simulink model "fw_att_control"  (R2021a)
settings: Solver=FixedStepAuto  StartTime=0.0  StopTime=10.0  RelTol=1e-3
undefined symbols (not defined in the file): DiscIntNeverNeededParam, FW_ACRO_X_MAX, FW_ACRO_Y_MAX, FW_ACRO_Z_MAX, FW_AIRSPD_MAX, FW_AIRSPD_STALL, FW_AIRSPD_TRIM, FW_BAT_SCALE_EN, FW_DTRIM_P_FLPS, FW_DTRIM_P_VMAX, FW_DTRIM_P_VMIN, FW_DTRIM_R_FLPS, FW_DTRIM_R_VMAX, FW_DTRIM_R_VMIN, FW_DTRIM_Y_VMAX, FW_DTRIM_Y_VMIN, FW_FLAPERON_SCL, FW_FLAPS_LND_SCL, FW_FLAPS_SCL, FW_FLAPS_TO_SCL, FW_MAN_P_MAX, FW_MAN_P_SC, FW_MAN_R_MAX, FW_MAN_R_SC, FW_MAN_Y_SC, FW_P_TC, FW_PR_IMAX, FW_PR_P, FW_PSP_OFF, FW_R_TC, FW_RLL_TO_YAW_FF, FW_RR_FF, FW_W_EN, FW_W_RMAX, FW_WR_FF, FW_WR_P, FW_Y_TC, FW_YR_FF, FW_YR_P, magnitude, PX4_VEHICLE_ATTITUDE_SETPOINT, PX4_VEHICLE_STATUS, TRIM_PITCH, TRIM_ROLL, TRIM_YAW
libraries: simulink x10, aerolibconvert2 x5, sharedtransform x2
(part 1 of 2)
settings Model: DataDictionary=px4_dict.sldd  Creator=DELL  LastModifiedBy=DELL
settings OptimizationCC: DefaultUnderspecifiedDataType=single

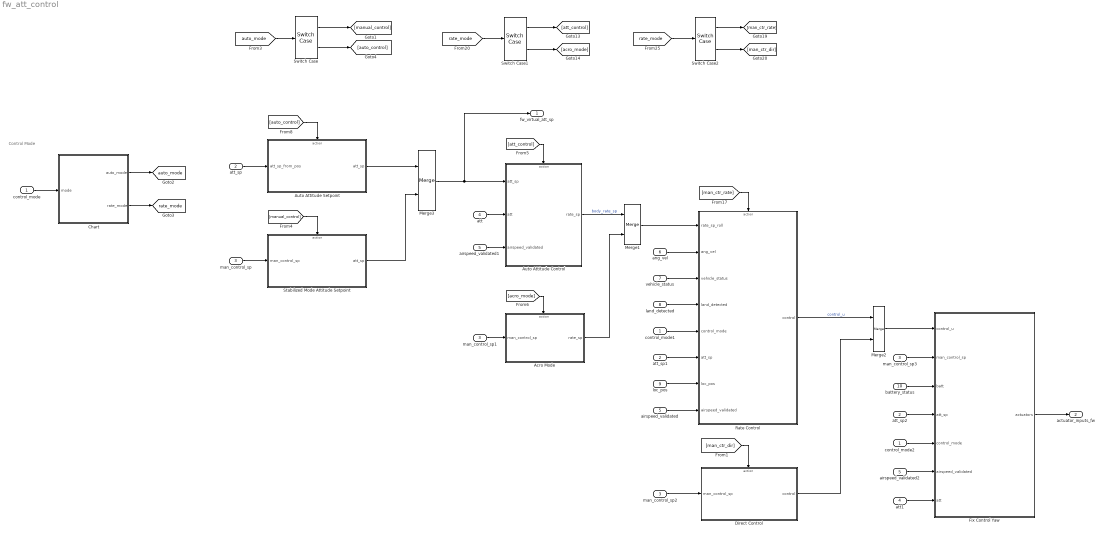
== system fw_att_control ==
  note: Control Mode
  control_mode : Inport  OutDataTypeStr=Bus: px4_vehicle_control_mode  BusOutputAsStruct=on
  att_sp : Inport  Port=2  OutDataTypeStr=Bus: px4_vehicle_attitude_setpoint  BusOutputAsStruct=on
  man_control_sp2 : Inport  Port=3  OutDataTypeStr=Bus: px4_manual_control_setpoint  BusOutputAsStruct=on
  att : Inport  Port=4  OutDataTypeStr=Bus: px4_vehicle_attitude  BusOutputAsStruct=on
  airspeed_validated1 : Inport  Port=5  OutDataTypeStr=Bus: px4_airspeed_validated  BusOutputAsStruct=on
  ang_vel : Inport  Port=6  OutDataTypeStr=Bus: px4_vehicle_angular_velocity  BusOutputAsStruct=on
  vehicle_status : Inport  Port=7  OutDataTypeStr=Bus: px4_vehicle_status  BusOutputAsStruct=on
  land_detected : Inport  Port=8  OutDataTypeStr=Bus: px4_vehicle_land_detected  BusOutputAsStruct=on
  loc_pos : Inport  Port=9  OutDataTypeStr=Bus: px4_vehicle_local_position
  battery_status : Inport  Port=10  OutDataTypeStr=Bus: px4_battery_status  BusOutputAsStruct=on
  Acro Mode : Subsystem  TreatAsAtomicUnit=on
  Auto Attitude Control : Subsystem
  Auto Attitude Setpoint : Subsystem
  Chart : Stateflow chart  TreatAsAtomicUnit=on
  "Direct Control " : Subsystem  TreatAsAtomicUnit=on
  Fix Control Yaw : Subsystem
  Merge1 : Merge
  Merge2 : Merge
  Merge3 : Merge
  Rate Control : Subsystem
  Stabilized Mode Attitude Setpoint : Subsystem  TreatAsAtomicUnit=on
  Switch Case : SwitchCase  CaseConditions={1,2 }  ShowDefaultCase=off
  Switch Case1 : SwitchCase  CaseConditions={1,2}  ShowDefaultCase=off
  Switch Case2 : SwitchCase  CaseConditions={2}
  airspeed_validated : InportShadow  Port=5  OutDataTypeStr=Bus: px4_airspeed_validated  BusOutputAsStruct=on
  airspeed_validated2 : InportShadow  Port=5  OutDataTypeStr=Bus: px4_airspeed_validated  BusOutputAsStruct=on
  att1 : InportShadow  Port=4  OutDataTypeStr=Bus: px4_vehicle_attitude  BusOutputAsStruct=on
  att_sp1 : InportShadow  Port=2  OutDataTypeStr=Bus: px4_vehicle_attitude_setpoint  BusOutputAsStruct=on
  att_sp2 : InportShadow  Port=2  OutDataTypeStr=Bus: px4_vehicle_attitude_setpoint  BusOutputAsStruct=on
  control_mode1 : InportShadow  OutDataTypeStr=Bus: px4_vehicle_control_mode  BusOutputAsStruct=on
  control_mode2 : InportShadow  OutDataTypeStr=Bus: px4_vehicle_control_mode  BusOutputAsStruct=on
  man_control_sp : InportShadow  Port=3  OutDataTypeStr=Bus: px4_manual_control_setpoint  BusOutputAsStruct=on
  man_control_sp1 : InportShadow  Port=3  OutDataTypeStr=Bus: px4_manual_control_setpoint  BusOutputAsStruct=on
  man_control_sp3 : InportShadow  Port=3  OutDataTypeStr=Bus: px4_manual_control_setpoint  BusOutputAsStruct=on
  fw_virtual_att_sp : Outport  OutDataTypeStr=Bus: px4_vehicle_attitude_setpoint  BusOutputAsStruct=on
  actuator_inputs_fw : Outport  Port=2  OutDataTypeStr=Bus: px4_actuator_controls_0  BusOutputAsStruct=on
  tag scope: auto_mode=global, rate_mode=global
  wires:
  Chart/1(auto_mode) -> [auto_mode]
  Chart/2(rate_mode) -> [rate_mode]
  control_mode/1 -> Chart/1(mode)
  att_sp2/1 -> Fix Control Yaw/4(att_sp)
  Auto Attitude Control/1(rate_sp) -> Merge1/1  "body_rate_sp"
  Acro Mode/1(rate_sp) -> Merge1/2
  [att_control] -> Auto Attitude Control/Action
  Switch Case1/2 -> [acro_mode]
  att/1 -> Auto Attitude Control/2(att)
  [rate_mode] -> Switch Case1/1
  Switch Case1/1 -> [att_control]
  man_control_sp1/1 -> Acro Mode/1(man_control_sp)
  Merge2/1 -> Fix Control Yaw/1(control_u)
  Rate Control/1(control) -> Merge2/1  "control_u"
  ang_vel/1 -> Rate Control/2(ang_vel)
  "Direct Control "/1(control) -> Merge2/2
  Switch Case2/2 -> [man_ctr_dir]
  [man_ctr_dir] -> "Direct Control "/Action
  [man_ctr_rate] -> Rate Control/Action
  Switch Case2/1 -> [man_ctr_rate]
  [rate_mode] -> Switch Case2/1
  man_control_sp2/1 -> "Direct Control "/1(man_control_sp)
  man_control_sp3/1 -> Fix Control Yaw/2(man_control_sp)
  control_mode2/1 -> Fix Control Yaw/5(control_mode)
  vehicle_status/1 -> Rate Control/3(vehicle_status)
  land_detected/1 -> Rate Control/4(land_detected)
  control_mode1/1 -> Rate Control/5(control_mode)
  att_sp1/1 -> Rate Control/6(att_sp)
  battery_status/1 -> Fix Control Yaw/3(batt)
  Merge1/1 -> Rate Control/1(rate_sp_roll)
  airspeed_validated2/1 -> Fix Control Yaw/6(airspeed_validated)
  airspeed_validated1/1 -> Auto Attitude Control/3(airspeed_validated)
  airspeed_validated/1 -> Rate Control/8(airspeed_validated)
  loc_pos/1 -> Rate Control/7(loc_pos)
  [auto_mode] -> Switch Case/1
  [acro_mode] -> Acro Mode/Action
  Switch Case/1 -> [manual_control]
  Switch Case/2 -> [auto_control]
  man_control_sp/1 -> Stabilized Mode Attitude Setpoint/1(man_control_sp)
  Merge3/1 -> fw_virtual_att_sp/1, Auto Attitude Control/1(att_sp)
  [manual_control] -> Stabilized Mode Attitude Setpoint/Action
  [auto_control] -> Auto Attitude Setpoint/Action
  att1/1 -> Fix Control Yaw/7(att)
  Fix Control Yaw/1(actuators) -> actuator_inputs_fw/1
  Stabilized Mode Attitude Setpoint/1(att_sp) -> Merge3/2
  Auto Attitude Setpoint/1(att_sp) -> Merge3/1
  att_sp/1 -> Auto Attitude Setpoint/1(att_sp_from_pos)

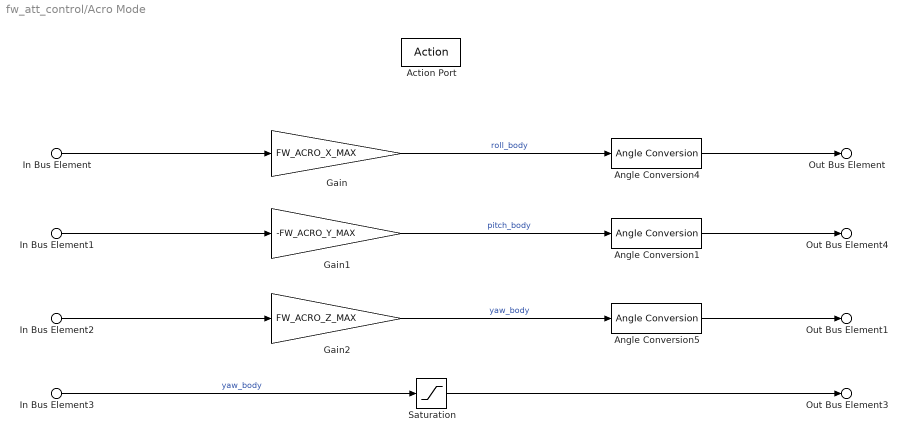
== system fw_att_control/Acro Mode ==
  In Bus Element : Inport  PortName=man_control_sp  Element=y
  In Bus Element1 : Inport  PortName=man_control_sp  Element=x
  In Bus Element2 : Inport  PortName=man_control_sp  Element=r
  In Bus Element3 : Inport  PortName=man_control_sp  Element=z
  Action Port : ActionPort  ActionPortLabel=case [ 2 ]:
  Angle Conversion1 : aerolibconvert2/Angle Conversion  IU=deg  OU=rad
  Angle Conversion4 : aerolibconvert2/Angle Conversion  IU=deg  OU=rad
  Angle Conversion5 : aerolibconvert2/Angle Conversion  IU=deg  OU=rad
  Gain : Gain  Gain=FW_ACRO_X_MAX
  Gain1 : Gain  Gain=-FW_ACRO_Y_MAX
  Gain2 : Gain  Gain=FW_ACRO_Z_MAX
  Saturation : Saturate  UpperLimit=1  LowerLimit=0
      settings: AttributesFormatString=[%<LowerLimit>,%<UpperLimit>]
  Out Bus Element : Outport  PortName=rate_sp  Element=roll
  Out Bus Element4 : Outport  PortName=rate_sp  Element=pitch
  Out Bus Element1 : Outport  PortName=rate_sp  Element=yaw
  Out Bus Element3 : Outport  PortName=rate_sp  Element=thrust
  wires:
  Gain1/1 -> Angle Conversion1/1  "pitch_body"
  In Bus Element3/1 -> Saturation/1  "yaw_body"
  Gain/1 -> Angle Conversion4/1  "roll_body"
  In Bus Element/1 -> Gain/1
  In Bus Element1/1 -> Gain1/1
  In Bus Element2/1 -> Gain2/1
  Gain2/1 -> Angle Conversion5/1  "yaw_body"
  Saturation/1 -> Out Bus Element3/1
  Angle Conversion4/1 -> Out Bus Element/1
  Angle Conversion1/1 -> Out Bus Element4/1
  Angle Conversion5/1 -> Out Bus Element1/1

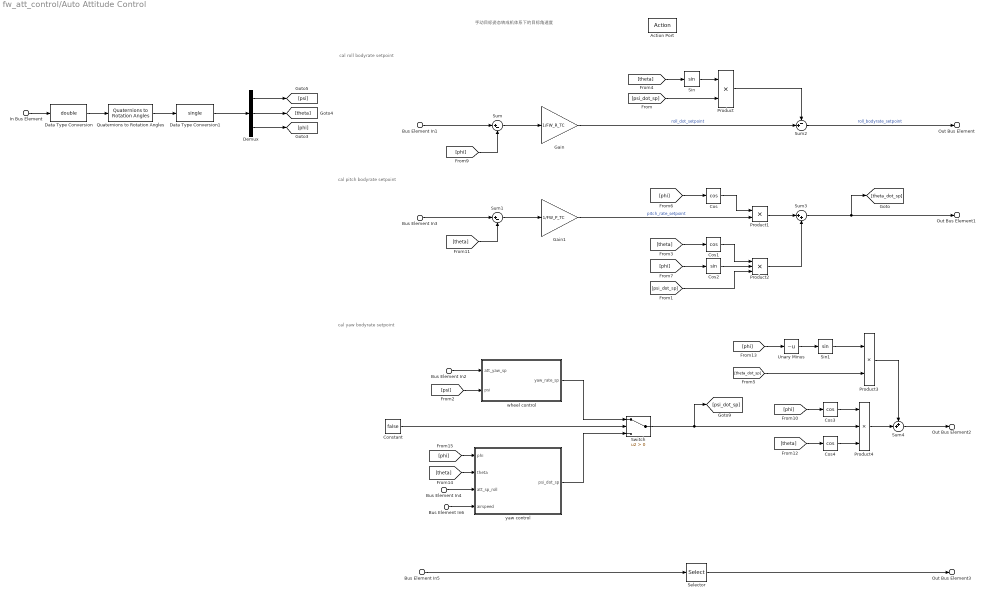
== system fw_att_control/Auto Attitude Control ==
  note: cal yaw bodyrate setpoint
  note: cal pitch bodyrate setpoint
  note: cal roll bodyrate setpoint
  note: 手动目标姿态转成机体系下的目标角速度
  Bus Element In3 : Inport  PortName=att_sp  Element=pitch_body
  Bus Element In5 : Inport  PortName=att_sp  Element=thrust_body
  Bus Element In2 : Inport  PortName=att_sp  Element=yaw_body
  Bus Element In1 : Inport  PortName=att_sp  Element=roll_body
  Bus Element In4 : Inport  PortName=att_sp  Element=roll_body
  In Bus Element : Inport  Port=2  PortName=att  Element=q
  Bus Element In6 : Inport  Port=3  PortName=airspeed_validated  Element=calibrated_airspeed_m_s
  Action Port : ActionPort  ActionPortLabel=case [ 1 ]:
  Constant : Constant  Value=false  OutDataTypeStr=boolean
  Cos{,1,3..4} (4 alike) : Trigonometry  Operator=cos
  Cos2 : Trigonometry
  Data Type Conversion : DataTypeConversion  OutDataTypeStr=double
  Data Type Conversion1 : DataTypeConversion  OutDataTypeStr=single
  Demux : Demux  Outputs=3
  Gain : Gain  Gain=1/FW_R_TC
  Gain1 : Gain  Gain=1/FW_P_TC
  Product : Product
  Product1 : Product
  Product2 : Product  Inputs=3
  Product3 : Product
  Product4 : Product  Inputs=3
  Quaternions to Rotation Angles : sharedtransform/Quaternions to Rotation Angles  rotationOrder=ZYX  aMode=aMode
      settings: SourceProductBaseCode=AE,PW,DR,MT,UV,VE
  Selector : Selector  InputPortWidth=3  IndexOptions=Index vector (dialog)  Indices=[1]  OutputSizes=1
  Sin : Trigonometry
  Sin1 : Trigonometry
  Sum : Sum  Inputs=|+-
  Sum1 : Sum  Inputs=|+-
  Sum2 : Sum  Inputs=-+|
  Sum3 : Sum  Inputs=|++
  Sum4 : Sum  Inputs=++|
  Switch : Switch  Criteria=u2 > Threshold
  Unary Minus : UnaryMinus
  wheel control : Subsystem  TreatAsAtomicUnit=on
  yaw control : Subsystem  TreatAsAtomicUnit=on
  Out Bus Element : Outport  PortName=rate_sp  Element=roll
  Out Bus Element1 : Outport  PortName=rate_sp  Element=pitch
  Out Bus Element2 : Outport  PortName=rate_sp  Element=yaw
  Out Bus Element3 : Outport  PortName=rate_sp  Element=thrust
  wires:
  Quaternions to Rotation Angles/1 -> Data Type Conversion1/1
  In Bus Element/1 -> Data Type Conversion/1
  Data Type Conversion/1 -> Quaternions to Rotation Angles/1
  Data Type Conversion1/1 -> Demux/1
  Demux/1 -> [psi]
  Demux/2 -> [theta]
  Demux/3 -> [phi]
  Sum3/1 -> Out Bus Element1/1, [theta_dot_sp]
  Sum2/1 -> Out Bus Element/1  "roll_bodyrate_setpoint"
  [theta] -> Sin/1
  Sin/1 -> Product/1
  Sum/1 -> Gain/1
  [phi] -> Sum/2
  [psi_dot_sp] -> Product/2
  Gain/1 -> Sum2/2  "roll_dot_setpoint"
  Bus Element In1/1 -> Sum/1
  Product/1 -> Sum2/1
  Bus Element In3/1 -> Sum1/1
  Cos1/1 -> Product2/1
  Cos/1 -> Product1/1
  Cos2/1 -> Product2/2
  Product2/1 -> Sum3/2
  Sum1/1 -> Gain1/1
  Product1/1 -> Sum3/1
  [theta] -> Cos1/1
  [psi_dot_sp] -> Product2/3
  [theta] -> Sum1/2
  [phi] -> Cos/1
  Gain1/1 -> Product1/2  "pitch_rate_setpoint"
  [phi] -> Cos2/1
  Bus Element In5/1 -> Selector/1
  [phi] -> Cos3/1
  [phi] -> Unary Minus/1
  Switch/1 -> Product4/2, [psi_dot_sp]
  Unary Minus/1 -> Sin1/1
  [theta_dot_sp] -> Product3/2
  Bus Element In4/1 -> yaw control/3(att_sp_roll)
  Bus Element In6/1 -> yaw control/4(airspeed)
  [psi] -> wheel control/2(psi)
  Bus Element In2/1 -> wheel control/1(att_yaw_sp)
  Sum4/1 -> Out Bus Element2/1
  Cos3/1 -> Product4/1
  Product3/1 -> Sum4/1
  Product4/1 -> Sum4/2
  Sin1/1 -> Product3/1
  [theta] -> Cos4/1
  Cos4/1 -> Product4/3
  [phi] -> yaw control/1(phi)
  [theta] -> yaw control/2(theta)
  wheel control/1(yaw_rate_sp) -> Switch/1
  yaw control/1(psi_dot_sp) -> Switch/3
  Constant/1 -> Switch/2
  Selector/1 -> Out Bus Element3/1

== system fw_att_control/Auto Attitude Setpoint ==
  att_sp_from_pos : Inport
  Action Port : ActionPort  ActionPortLabel=case [ 2 ]:
  Signal Conversion : SignalConversion  ConversionOutput=Virtual bus  OverrideOpt=off
  att_sp : Outport
  wires:
  att_sp_from_pos/1 -> Signal Conversion/1
  Signal Conversion/1 -> att_sp/1

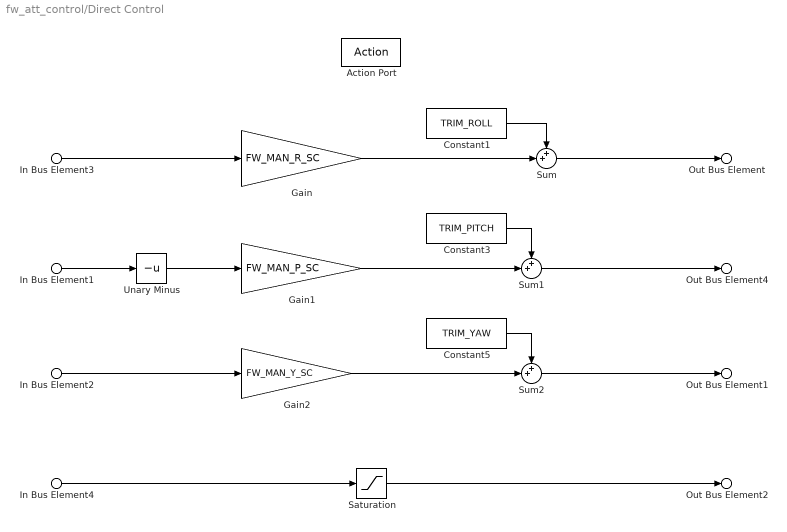
== system fw_att_control/Direct Control  ==
  In Bus Element3 : Inport  PortName=man_control_sp  Element=y
  In Bus Element1 : Inport  PortName=man_control_sp  Element=x
  In Bus Element2 : Inport  PortName=man_control_sp  Element=r
  In Bus Element4 : Inport  PortName=man_control_sp  Element=z
  Action Port : ActionPort  ActionPortLabel=default:
  Constant1 : Constant  Value=TRIM_ROLL
  Constant3 : Constant  Value=TRIM_PITCH
  Constant5 : Constant  Value=TRIM_YAW
  Gain : Gain  Gain=FW_MAN_R_SC
  Gain1 : Gain  Gain=FW_MAN_P_SC
  Gain2 : Gain  Gain=FW_MAN_Y_SC
  Saturation : Saturate  UpperLimit=1  LowerLimit=0
      settings: AttributesFormatString=[%<LowerLimit>,%<UpperLimit>]
  Sum : Sum  Inputs=++|
  Sum1 : Sum  Inputs=++|
  Sum2 : Sum  Inputs=++|
  Unary Minus : UnaryMinus
  Out Bus Element : Outport  PortName=control  Element=index_roll
  Out Bus Element4 : Outport  PortName=control  Element=index_pitch
  Out Bus Element1 : Outport  PortName=control  Element=index_yaw
  Out Bus Element2 : Outport  PortName=control  Element=index_throttle
  wires:
  In Bus Element3/1 -> Gain/1
  Sum/1 -> Out Bus Element/1
  Sum1/1 -> Out Bus Element4/1
  In Bus Element1/1 -> Unary Minus/1
  Unary Minus/1 -> Gain1/1
  In Bus Element2/1 -> Gain2/1
  Sum2/1 -> Out Bus Element1/1
  In Bus Element4/1 -> Saturation/1
  Saturation/1 -> Out Bus Element2/1
  Constant1/1 -> Sum/1
  Gain/1 -> Sum/2
  Constant3/1 -> Sum1/1
  Gain1/1 -> Sum1/2
  Constant5/1 -> Sum2/1
  Gain2/1 -> Sum2/2

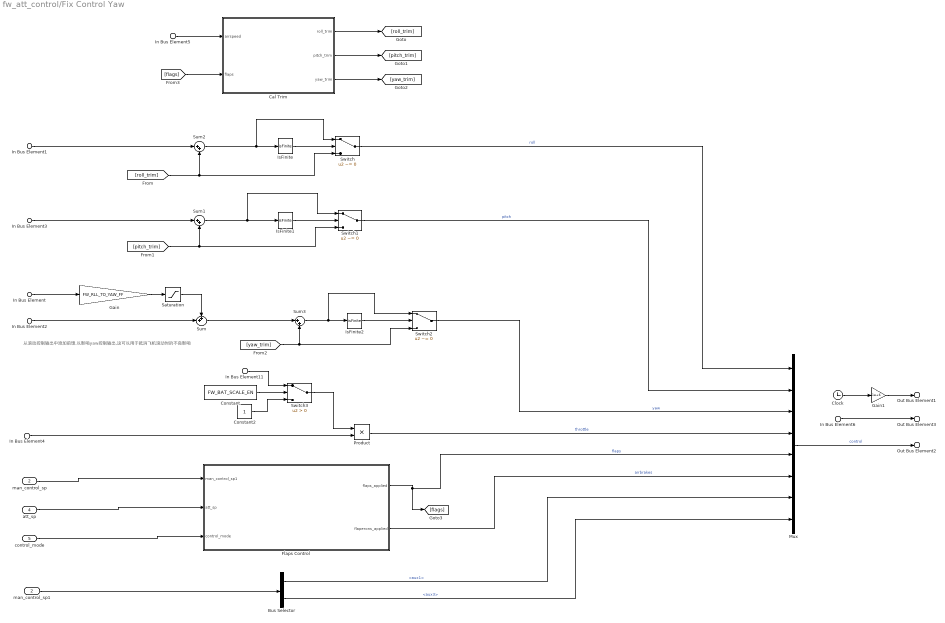
== system fw_att_control/Fix Control Yaw ==
  note: 从滚动控制输出中添加前馈,以影响yaw控制输出,这可以用于抵消飞机滚动时的不良影响
  In Bus Element1 : Inport  PortName=control_u  Element=index_roll
  In Bus Element : Inport  PortName=control_u  Element=index_roll
  In Bus Element3 : Inport  PortName=control_u  Element=index_pitch
  In Bus Element2 : Inport  PortName=control_u  Element=index_yaw
  In Bus Element4 : Inport  PortName=control_u  Element=index_throttle
  man_control_sp : Inport  Port=2
  In Bus Element11 : Inport  Port=3  PortName=batt  Element=scale
  att_sp : Inport  Port=4
  control_mode : Inport  Port=5
  In Bus Element5 : Inport  Port=6  PortName=airspeed_validated  Element=calibrated_airspeed_m_s
  In Bus Element6 : Inport  Port=7  PortName=att  Element=timestamp
  Bus Selector : BusSelector  OutputSignals=aux1,aux3
  Cal Trim : Subsystem
  Clock : Clock
  Constant : Constant  Value=FW_BAT_SCALE_EN  OutDataTypeStr=boolean
  Constant2 : Constant  OutDataTypeStr=single
  Flaps Control : Subsystem
  Gain : Gain  Gain=FW_RLL_TO_YAW_FF
  Gain1 : Gain  Gain=1e+6  OutDataTypeStr=uint64
      settings: AttributesFormatString=%<Gain>
  IsFinite : RelationalOperator  Operator=isFinite  OutDataTypeStr=boolean  RndMeth=Simplest
  IsFinite1 : RelationalOperator  Operator=isFinite  OutDataTypeStr=boolean  RndMeth=Simplest
  IsFinite2 : RelationalOperator  Operator=isFinite  OutDataTypeStr=boolean  RndMeth=Simplest
  Mux : Mux  Inputs=8
  Product : Product
  Saturation : Saturate  UpperLimit=1  LowerLimit=-1
      settings: AttributesFormatString=[%<LowerLimit>,%<UpperLimit>]
  Sum : Sum  Inputs=++|
  Sum1 : Sum  Inputs=|++
  Sum2 : Sum  Inputs=|++
  Sum3 : Sum  Inputs=|++
  Switch : Switch  Criteria=u2 ~= 0
  Switch1 : Switch  Criteria=u2 ~= 0
  Switch2 : Switch  Criteria=u2 ~= 0
  Switch3 : Switch  Criteria=u2 > Threshold
  man_control_sp1 : InportShadow  Port=2
  Out Bus Element1 : Outport  PortName=actuators  Element=timestamp
  Out Bus Element3 : Outport  PortName=actuators  Element=timestamp_sample
  Out Bus Element2 : Outport  PortName=actuators  Element=control
  wires:
  In Bus Element/1 -> Gain/1
  Saturation/1 -> Sum/1
  In Bus Element2/1 -> Sum/2
  Product/1 -> Mux/4  "throttle"
  control_mode/1 -> Flaps Control/3(control_mode)
  att_sp/1 -> Flaps Control/2(att_sp)
  Bus Selector/1 -> Mux/7  "<aux1>"
  Bus Selector/2 -> Mux/8  "<aux3>"
  Flaps Control/2(flaperons_applied) -> Mux/6  "airbrakes"
  man_control_sp/1 -> Flaps Control/1(man_control_sp1)
  Flaps Control/1(flaps_applied) -> Mux/5, [flags]  "flaps"
  man_control_sp1/1 -> Bus Selector/1
  In Bus Element4/1 -> Product/2
  In Bus Element1/1 -> Sum2/1
  Sum2/1 -> Switch/1, IsFinite/1
  IsFinite/1 -> Switch/2
  Switch/1 -> Mux/1  "roll"
  Switch1/1 -> Mux/2  "pitch"
  IsFinite1/1 -> Switch1/2
  IsFinite2/1 -> Switch2/2
  Switch2/1 -> Mux/3  "yaw"
  Sum/1 -> Sum3/1
  In Bus Element11/1 -> Switch3/1
  Constant/1 -> Switch3/2
  Switch3/1 -> Product/1
  Constant2/1 -> Switch3/3
  Sum1/1 -> Switch1/1, IsFinite1/1
  Sum3/1 -> Switch2/1, IsFinite2/1
  Cal Trim/1(roll_trim) -> [roll_trim]
  In Bus Element3/1 -> Sum1/1
  Cal Trim/2(pitch_trim) -> [pitch_trim]
  Cal Trim/3(yaw_trim) -> [yaw_trim]
  [pitch_trim] -> Switch1/3, Sum1/2
  [roll_trim] -> Sum2/2, Switch/3
  [yaw_trim] -> Sum3/2, Switch2/3
  [flags] -> Cal Trim/2(flaps)
  In Bus Element5/1 -> Cal Trim/1(airspeed)
  Gain/1 -> Saturation/1
  Clock/1 -> Gain1/1
  Gain1/1 -> Out Bus Element1/1
  Mux/1 -> Out Bus Element2/1  "control"
  In Bus Element6/1 -> Out Bus Element3/1

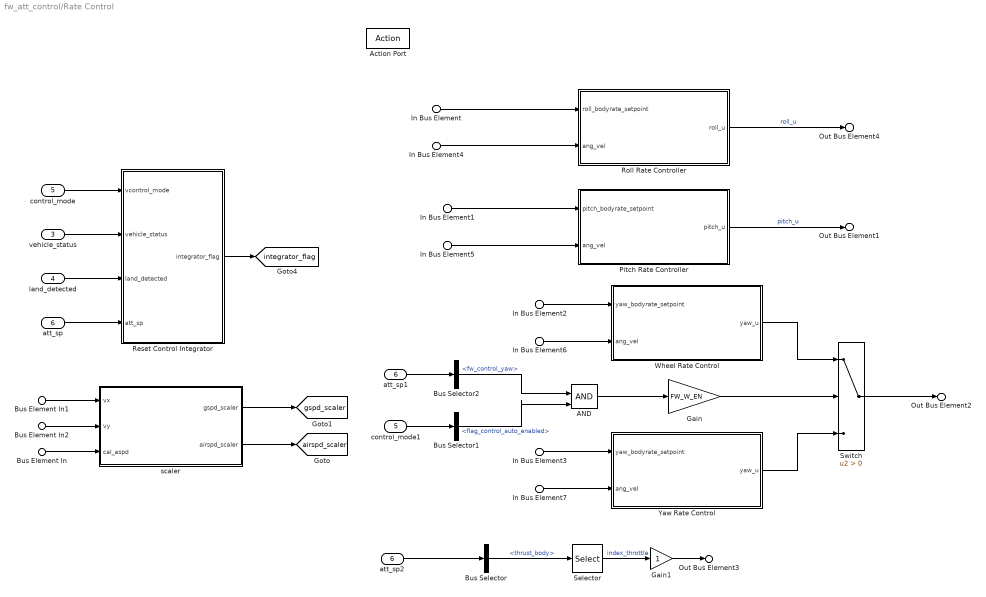
== system fw_att_control/Rate Control ==
  In Bus Element : Inport  PortName=rate_sp_roll  Element=roll
  In Bus Element1 : Inport  PortName=rate_sp_roll  Element=pitch
  In Bus Element2 : Inport  PortName=rate_sp_roll  Element=yaw
  In Bus Element3 : Inport  PortName=rate_sp_roll  Element=yaw
  In Bus Element{4..7} (4 alike) : Inport  Port=2  PortName=ang_vel  Element=xyz
  vehicle_status : Inport  Port=3  OutDataTypeStr=Bus: px4_vehicle_status
  land_detected : Inport  Port=4  OutDataTypeStr=Bus: px4_vehicle_land_detected
  control_mode : Inport  Port=5  OutDataTypeStr=Bus: px4_vehicle_control_mode
  att_sp : Inport  Port=6
  Bus Element In1 : Inport  Port=7  PortName=loc_pos  Element=vx
  Bus Element In2 : Inport  Port=7  PortName=loc_pos  Element=vy
  Bus Element In : Inport  Port=8  PortName=airspeed_validated  Element=calibrated_airspeed_m_s
  Action Port : ActionPort  ActionPortLabel=case [ 2 ]:
  AND : Logic  IconShape=distinctive  AllPortsSameDT=off  OutDataTypeStr=boolean
  Bus Selector : BusSelector  OutputSignals=thrust_body
  Bus Selector1 : BusSelector  OutputSignals=flag_control_auto_enabled
  Bus Selector2 : BusSelector  OutputSignals=fw_control_yaw
  Gain : Gain  Gain=FW_W_EN
  Gain1 : Gain
  Pitch Rate Controller : Subsystem
  Reset Control Integrator : Subsystem
  Roll Rate Controller : Subsystem
  Selector : Selector  InputPortWidth=3  IndexOptions=Index vector (dialog)  Indices=[1]  OutputSizes=1
  Switch : Switch  Criteria=u2 > Threshold
  Wheel Rate Control : Subsystem
  Yaw Rate Control : Subsystem
  att_sp1 : InportShadow  Port=6
  att_sp2 : InportShadow  Port=6
  control_mode1 : InportShadow  Port=5  OutDataTypeStr=Bus: px4_vehicle_control_mode
  scaler : Subsystem
  Out Bus Element4 : Outport  PortName=control  Element=index_roll
  Out Bus Element1 : Outport  PortName=control  Element=index_pitch
  Out Bus Element2 : Outport  PortName=control  Element=index_yaw
  Out Bus Element3 : Outport  PortName=control  Element=index_throttle
  tag scope: airspd_scaler=global, gspd_scaler=global, integrator_flag=global
  wires:
  In Bus Element/1 -> Roll Rate Controller/1(roll_bodyrate_setpoint)
  In Bus Element1/1 -> Pitch Rate Controller/1(pitch_bodyrate_setpoint)
  In Bus Element5/1 -> Pitch Rate Controller/2(ang_vel)
  Selector/1 -> Gain1/1  "index_throttle"
  vehicle_status/1 -> Reset Control Integrator/2(vehicle_status)
  land_detected/1 -> Reset Control Integrator/3(land_detected)
  control_mode/1 -> Reset Control Integrator/1(vcontrol_mode)
  att_sp/1 -> Reset Control Integrator/4(att_sp)
  Reset Control Integrator/1(integrator_flag) -> [integrator_flag]
  Roll Rate Controller/1(roll_u) -> Out Bus Element4/1  "roll_u"
  Pitch Rate Controller/1(pitch_u) -> Out Bus Element1/1  "pitch_u"
  Switch/1 -> Out Bus Element2/1
  AND/1 -> Gain/1
  In Bus Element6/1 -> Wheel Rate Control/2(ang_vel)
  In Bus Element2/1 -> Wheel Rate Control/1(yaw_bodyrate_setpoint)
  Wheel Rate Control/1(yaw_u) -> Switch/1
  In Bus Element3/1 -> Yaw Rate Control/1(yaw_bodyrate_setpoint)
  In Bus Element7/1 -> Yaw Rate Control/2(ang_vel)
  Yaw Rate Control/1(yaw_u) -> Switch/3
  In Bus Element4/1 -> Roll Rate Controller/2(ang_vel)
  Bus Element In2/1 -> scaler/2(vy)
  Bus Element In1/1 -> scaler/1(vx)
  Bus Element In/1 -> scaler/3(cal_aspd)
  scaler/2(airspd_scaler) -> [airspd_scaler]
  scaler/1(gspd_scaler) -> [gspd_scaler]
  Bus Selector/1 -> Selector/1  "<thrust_body>"
  att_sp2/1 -> Bus Selector/1
  Gain/1 -> Switch/2
  control_mode1/1 -> Bus Selector1/1
  Bus Selector1/1 -> AND/2  "<flag_control_auto_enabled>"
  att_sp1/1 -> Bus Selector2/1
  Bus Selector2/1 -> AND/1  "<fw_control_yaw>"
  Gain1/1 -> Out Bus Element3/1

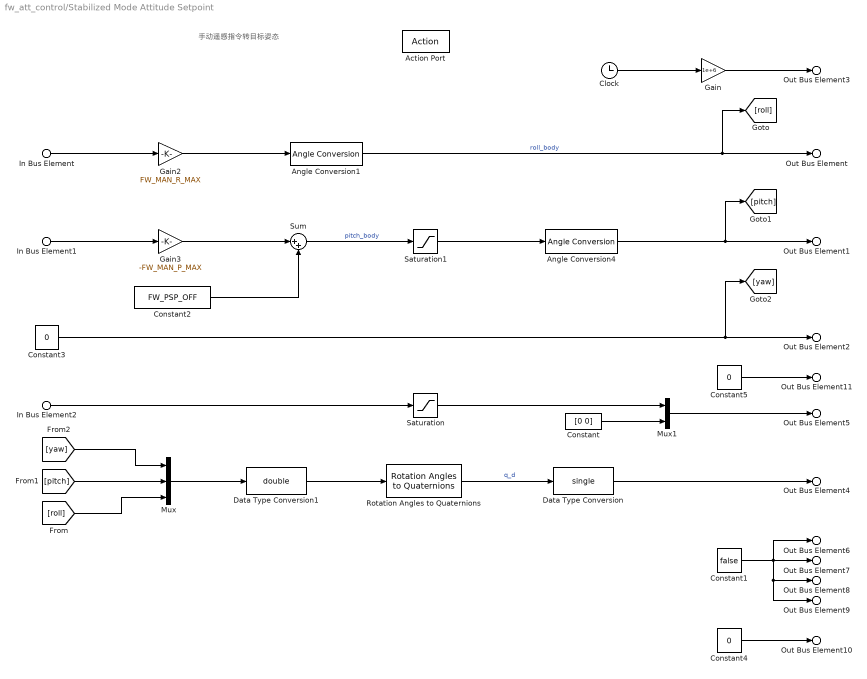
== system fw_att_control/Stabilized Mode Attitude Setpoint ==
  note: 手动遥感指令转目标姿态
  In Bus Element : Inport  PortName=man_control_sp  Element=y
  In Bus Element1 : Inport  PortName=man_control_sp  Element=x
  In Bus Element2 : Inport  PortName=man_control_sp  Element=z
  Action Port : ActionPort  ActionPortLabel=case [ 1 ]:
  Angle Conversion1 : aerolibconvert2/Angle Conversion  IU=deg  OU=rad
  Angle Conversion4 : aerolibconvert2/Angle Conversion  IU=deg  OU=rad
  Clock : Clock
  Constant : Constant  Value=[0 0]  OutDataTypeStr=single
  Constant1 : Constant  Value=false  OutDataTypeStr=boolean
  Constant2 : Constant  Value=FW_PSP_OFF
  Constant3 : Constant  Value=0  OutDataTypeStr=single
  Constant4 : Constant  Value=0  OutDataTypeStr=uint8
  Constant5 : Constant  Value=0  OutDataTypeStr=single
  Data Type Conversion : DataTypeConversion  OutDataTypeStr=single
  Data Type Conversion1 : DataTypeConversion  OutDataTypeStr=double
  Gain : Gain  Gain=1e+6  OutDataTypeStr=uint64
      settings: AttributesFormatString=%<Gain>
  Gain2 : Gain  Gain=FW_MAN_R_MAX
      settings: AttributesFormatString=%<Gain>
  Gain3 : Gain  Gain=-FW_MAN_P_MAX
      settings: AttributesFormatString=%<Gain>
  Mux : Mux  Inputs=3
  Mux1 : Mux  Inputs=2
  Rotation Angles to Quaternions : sharedtransform/Rotation Angles to Quaternions  rotationOrder=ZYX  aMode=aMode
      settings: SourceProductBaseCode=AE,PW,DR,MT,UV,VE
  Saturation : Saturate  UpperLimit=1.0  LowerLimit=0.0
      settings: AttributesFormatString=[%<LowerLimit>, %<UpperLimit>]
  Saturation1 : Saturate  UpperLimit=FW_MAN_P_MAX  LowerLimit=-FW_MAN_P_MAX
      settings: AttributesFormatString=[%<LowerLimit>, %<UpperLimit>]
  Sum : Sum  Inputs=|++
  Out Bus Element3 : Outport  PortName=att_sp  Element=timestamp
  Out Bus Element : Outport  PortName=att_sp  Element=roll_body
  Out Bus Element1 : Outport  PortName=att_sp  Element=pitch_body
  Out Bus Element2 : Outport  PortName=att_sp  Element=yaw_body
  Out Bus Element11 : Outport  PortName=att_sp  Element=yaw_sp_move_rate
  Out Bus Element4 : Outport  PortName=att_sp  Element=q_d
  Out Bus Element5 : Outport  PortName=att_sp  Element=thrust_body
  Out Bus Element6 : Outport  PortName=att_sp  Element=roll_reset_integral
  Out Bus Element7 : Outport  PortName=att_sp  Element=pitch_reset_integral
  Out Bus Element8 : Outport  PortName=att_sp  Element=yaw_reset_integral
  Out Bus Element9 : Outport  PortName=att_sp  Element=fw_control_yaw
  Out Bus Element10 : Outport  PortName=att_sp  Element=apply_flaps
  wires:
  Angle Conversion1/1 -> Out Bus Element/1, [roll]  "roll_body"
  In Bus Element/1 -> Gain2/1
  Gain2/1 -> Angle Conversion1/1
  Sum/1 -> Saturation1/1  "pitch_body"
  Saturation1/1 -> Angle Conversion4/1
  Constant2/1 -> Sum/2
  Gain3/1 -> Sum/1
  In Bus Element1/1 -> Gain3/1
  Angle Conversion4/1 -> Out Bus Element1/1, [pitch]
  Constant3/1 -> [yaw], Out Bus Element2/1
  Rotation Angles to Quaternions/1 -> Data Type Conversion/1  "q_d"
  Data Type Conversion/1 -> Out Bus Element4/1
  [pitch] -> Mux/2
  Data Type Conversion1/1 -> Rotation Angles to Quaternions/1
  Mux/1 -> Data Type Conversion1/1
  [roll] -> Mux/3
  [yaw] -> Mux/1
  In Bus Element2/1 -> Saturation/1
  Clock/1 -> Gain/1
  Gain/1 -> Out Bus Element3/1
  Constant1/1 -> Out Bus Element7/1, Out Bus Element6/1, Out Bus Element9/1, Out Bus Element8/1
  Constant4/1 -> Out Bus Element10/1
  Saturation/1 -> Mux1/1
  Constant/1 -> Mux1/2
  Mux1/1 -> Out Bus Element5/1
  Constant5/1 -> Out Bus Element11/1

== system fw_att_control/Auto Attitude Control/wheel control ==
  att_yaw_sp : Inport
  psi : Inport  Port=2
  Saturation1 : Saturate  UpperLimit=FW_W_RMAX  LowerLimit=-FW_W_RMAX
      settings: AttributesFormatString=[%<LowerLimit>,%<UpperLimit>]
  Sum : Sum  Inputs=|+-
  Wrap -pi~pi : Subsystem
  gain : Gain  Gain=1/FW_Y_TC
  yaw_rate_sp : Outport
  wires:
  att_yaw_sp/1 -> Sum/1
  psi/1 -> Sum/2
  gain/1 -> Saturation1/1
  Saturation1/1 -> yaw_rate_sp/1  "wheel_rate_setpoint"
  Sum/1 -> Wrap -pi~pi/1(In1)
  Wrap -pi~pi/1(Out1) -> gain/1

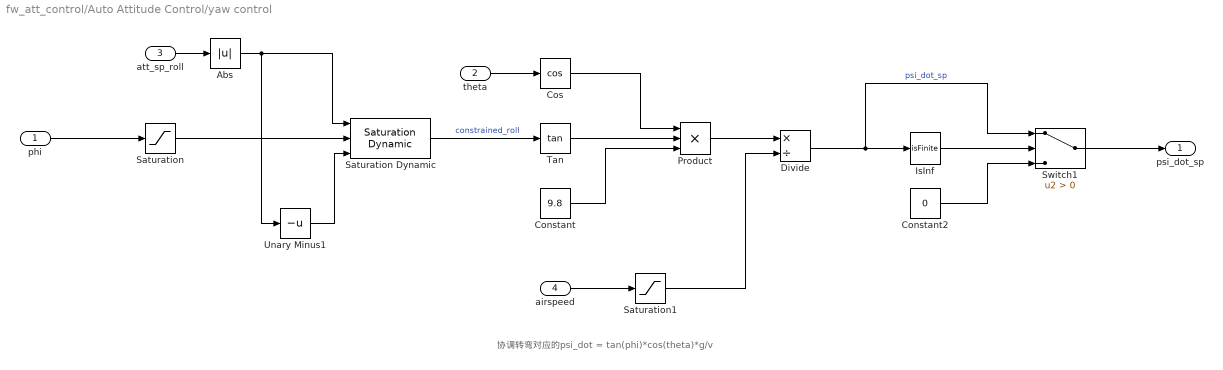
== system fw_att_control/Auto Attitude Control/yaw control ==
  note: 协调转弯对应的psi_dot = tan(phi)*cos(theta)*g/v
  phi : Inport
  theta : Inport  Port=2
  att_sp_roll : Inport  Port=3
  airspeed : Inport  Port=4
  Abs : Abs
  Constant : Constant  Value=9.8
  Constant2 : Constant  Value=0  OutDataTypeStr=single
  Cos : Trigonometry  Operator=cos
  Divide : Product  Inputs=*/
  IsInf : RelationalOperator  Operator=isFinite  OutDataTypeStr=boolean  RndMeth=Simplest
  Product : Product  Inputs=3
  Saturation : Saturate  UpperLimit=80*pi/180  LowerLimit=-80*pi/180
      settings: AttributesFormatString=[%<LowerLimit>,%<UpperLimit>]
  Saturation Dynamic : simulink/Discontinuities/Saturation Dynamic  OutMin=[]  OutMax=[]  OutDataTypeStr=Inherit: Same as second input  OutDataType=fixdt(1, 16)  OutScaling=2^-10  DoSatur=off
  Saturation1 : Saturate  UpperLimit=inf  LowerLimit=FW_AIRSPD_STALL
      settings: AttributesFormatString=[%<LowerLimit>,%<UpperLimit>]
  Switch1 : Switch  Criteria=u2 > Threshold
  Tan : Trigonometry  Operator=tan
  Unary Minus1 : UnaryMinus
  psi_dot_sp : Outport
  wires:
  Divide/1 -> Switch1/1, IsInf/1  "psi_dot_sp"
  phi/1 -> Saturation/1
  Saturation/1 -> Saturation Dynamic/2
  Abs/1 -> Saturation Dynamic/1, Unary Minus1/1
  Unary Minus1/1 -> Saturation Dynamic/3
  Saturation Dynamic/1 -> Tan/1  "constrained_roll"
  Tan/1 -> Product/2
  Cos/1 -> Product/1
  theta/1 -> Cos/1
  Constant/1 -> Product/3
  Product/1 -> Divide/1
  Saturation1/1 -> Divide/2
  att_sp_roll/1 -> Abs/1
  IsInf/1 -> Switch1/2
  Switch1/1 -> psi_dot_sp/1
  Constant2/1 -> Switch1/3
  airspeed/1 -> Saturation1/1

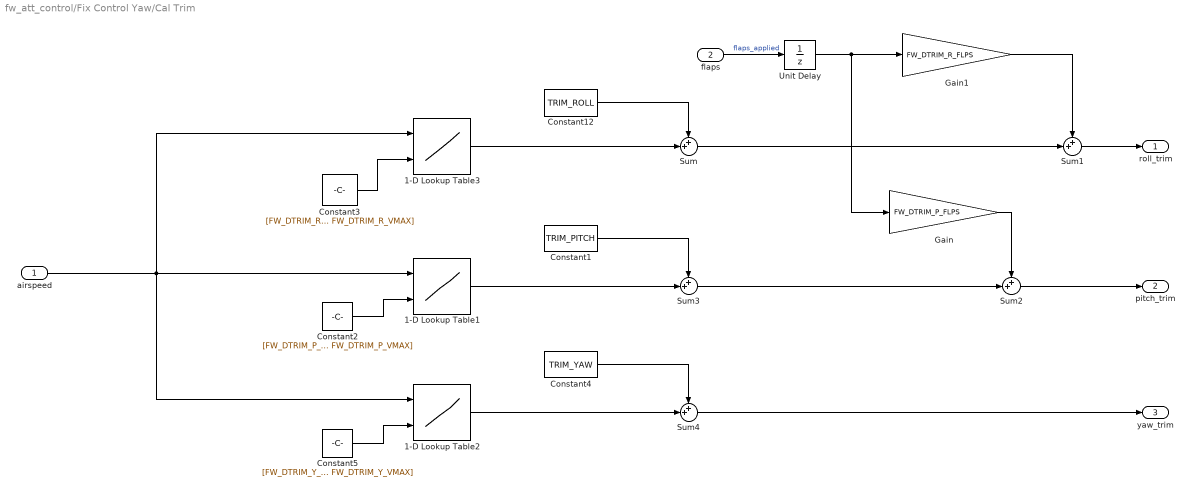
== system fw_att_control/Fix Control Yaw/Cal Trim ==
  airspeed : Inport
  flaps : Inport  Port=2
  1-D Lookup Table1 : Lookup_n-D  NumberOfTableDimensions=1  BreakpointsForDimension1=[FW_AIRSPD_STALL FW_AIRSPD_TRIM FW_AIRSPD_MAX]  TableSource=Input port  Table=tanh([-5:5])  ExtrapMethod=Clip  InternalRulePriority=Speed  RndMeth=Simplest  InputSameDT=on
      settings: InputPortMap=u0,p221
  1-D Lookup Table2 : Lookup_n-D  NumberOfTableDimensions=1  BreakpointsForDimension1=[FW_AIRSPD_STALL FW_AIRSPD_TRIM FW_AIRSPD_MAX]  TableSource=Input port  Table=tanh([-5:5])  ExtrapMethod=Clip  InternalRulePriority=Speed  RndMeth=Simplest  InputSameDT=on
      settings: InputPortMap=u0,p221
  1-D Lookup Table3 : Lookup_n-D  NumberOfTableDimensions=1  BreakpointsForDimension1=[FW_AIRSPD_STALL FW_AIRSPD_TRIM FW_AIRSPD_MAX]  TableSource=Input port  Table=tanh([-5:5])  ExtrapMethod=Clip  InternalRulePriority=Speed  RndMeth=Simplest  InputSameDT=on
      settings: InputPortMap=u0,p221
  Constant1 : Constant  Value=TRIM_PITCH
  Constant12 : Constant  Value=TRIM_ROLL
  Constant2 : Constant  Value=[FW_DTRIM_P_VMIN 0 FW_DTRIM_P_VMAX]
      settings: AttributesFormatString=%<Value>
  Constant3 : Constant  Value=[FW_DTRIM_R_VMIN 0 FW_DTRIM_R_VMAX]
      settings: AttributesFormatString=%<Value>
  Constant4 : Constant  Value=TRIM_YAW
  Constant5 : Constant  Value=[FW_DTRIM_Y_VMIN 0 FW_DTRIM_Y_VMAX]
      settings: AttributesFormatString=%<Value>
  Gain : Gain  Gain=FW_DTRIM_P_FLPS
  Gain1 : Gain  Gain=FW_DTRIM_R_FLPS
  Sum{,1..4} (5 alike) : Sum  Inputs=++|
  Unit Delay : UnitDelay  SampleTime=-1  HasFrameUpgradeWarning=on
  roll_trim : Outport
  pitch_trim : Outport  Port=2
  yaw_trim : Outport  Port=3
  wires:
  flaps/1 -> Unit Delay/1  "flaps_applied"
  Sum1/1 -> roll_trim/1
  Sum2/1 -> pitch_trim/1
  Gain/1 -> Sum2/1
  Gain1/1 -> Sum1/1
  Unit Delay/1 -> Gain/1, Gain1/1
  Constant3/1 -> 1-D Lookup Table3/2
  Sum/1 -> Sum1/2
  1-D Lookup Table3/1 -> Sum/2
  Constant12/1 -> Sum/1
  Constant1/1 -> Sum3/1
  1-D Lookup Table1/1 -> Sum3/2
  Sum3/1 -> Sum2/2
  airspeed/1 -> 1-D Lookup Table2/1, 1-D Lookup Table3/1, 1-D Lookup Table1/1
  Constant2/1 -> 1-D Lookup Table1/2
  Constant5/1 -> 1-D Lookup Table2/2
  Sum4/1 -> yaw_trim/1
  1-D Lookup Table2/1 -> Sum4/2
  Constant4/1 -> Sum4/1

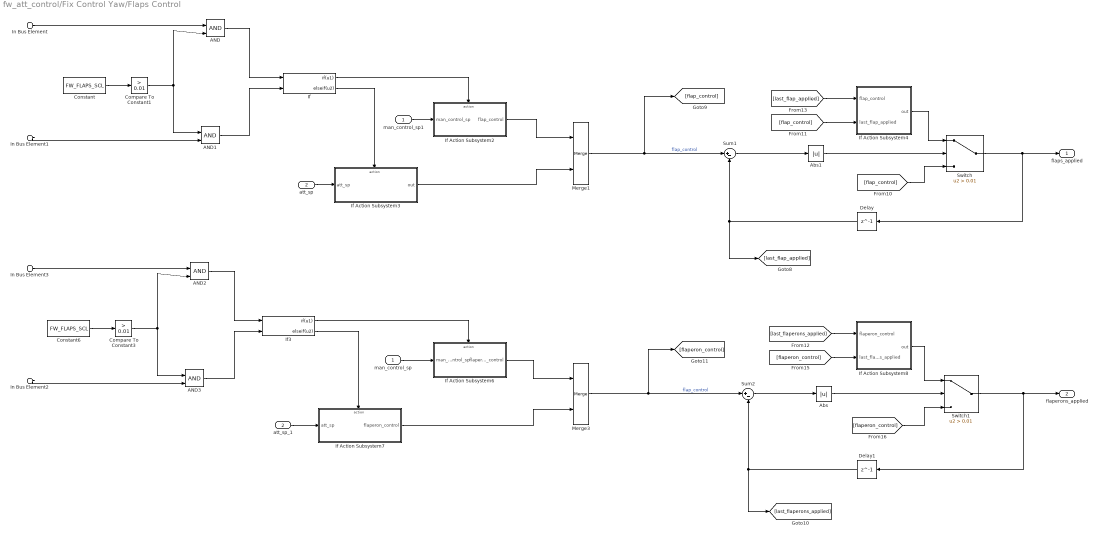
== system fw_att_control/Fix Control Yaw/Flaps Control ==
  man_control_sp1 : Inport  OutDataTypeStr=Bus: px4_manual_control_setpoint
  att_sp : Inport  Port=2  OutDataTypeStr=Bus: px4_vehicle_attitude_setpoint
  In Bus Element : Inport  Port=3  PortName=control_mode  Element=flag_control_manual_enabled
  In Bus Element3 : Inport  Port=3  PortName=control_mode  Element=flag_control_manual_enabled
  In Bus Element1 : Inport  Port=3  PortName=control_mode  Element=flag_control_auto_enabled
  In Bus Element2 : Inport  Port=3  PortName=control_mode  Element=flag_control_auto_enabled
  AND{,1..3} (4 alike) : Logic  IconShape=distinctive  AllPortsSameDT=off  OutDataTypeStr=boolean
  Abs : Abs
  Abs1 : Abs
  Compare To Constant1 : simulink/Logic and Bit Operations/Compare To Constant  relop=>  const=0.01  OutDataTypeStr=boolean
  Compare To Constant3 : simulink/Logic and Bit Operations/Compare To Constant  relop=>  const=0.01  OutDataTypeStr=boolean
  Constant : Constant  Value=FW_FLAPS_SCL  OutDataTypeStr=single
  Constant6 : Constant  Value=FW_FLAPS_SCL
  Delay : Delay  DelayLength=1
  Delay1 : Delay  DelayLength=1
  If : If  NumInputs=2  IfExpression=u1  ElseIfExpressions=u2  ShowElse=off
  If Action Subsystem2 : Subsystem  TreatAsAtomicUnit=on
  If Action Subsystem3 : Subsystem  TreatAsAtomicUnit=on
  If Action Subsystem4 : Subsystem  TreatAsAtomicUnit=on
  If Action Subsystem6 : Subsystem  TreatAsAtomicUnit=on
  If Action Subsystem7 : Subsystem  TreatAsAtomicUnit=on
  If Action Subsystem8 : Subsystem  TreatAsAtomicUnit=on
  If3 : If  NumInputs=2  IfExpression=u1  ElseIfExpressions=u2  ShowElse=off
  Merge1 : Merge
  Merge3 : Merge
  Sum1 : Sum  Inputs=|+-
  Sum2 : Sum  Inputs=|+-
  Switch : Switch  Criteria=u2 > Threshold  Threshold=0.01
  Switch1 : Switch  Criteria=u2 > Threshold  Threshold=0.01
  att_sp_1 : InportShadow  Port=2  OutDataTypeStr=Bus: px4_vehicle_attitude_setpoint
  man_control_sp : InportShadow  OutDataTypeStr=Bus: px4_manual_control_setpoint
  flaps_applied : Outport
  flaperons_applied : Outport  Port=2
  wires:
  Delay/1 -> [last_flap_applied], Sum1/2
  If Action Subsystem3/1(out) -> Merge1/2
  Delay1/1 -> [last_flaperons_applied], Sum2/2
  Constant/1 -> Compare To Constant1/1
  If Action Subsystem7/1(flaperon_control) -> Merge3/2
  Sum2/1 -> Abs/1
  If3/1 -> If Action Subsystem6/Action
  Compare To Constant1/1 -> AND/2, AND1/1
  att_sp/1 -> If Action Subsystem3/1(att_sp)
  If Action Subsystem6/1(flaperon_control) -> Merge3/1
  Compare To Constant3/1 -> AND2/2, AND3/1
  Merge1/1 -> Sum1/1, [flap_control]  "flap_control"
  man_control_sp/1 -> If Action Subsystem6/1(man_control_sp)
  Sum1/1 -> Abs1/1
  Merge3/1 -> Sum2/1, [flaperon_control]  "flap_control"
  If3/2 -> If Action Subsystem7/Action
  man_control_sp1/1 -> If Action Subsystem2/1(man_control_sp)
  [flaperon_control] -> If Action Subsystem8/2(last_flaperons_applied)
  If Action Subsystem2/1(flap_control) -> Merge1/1
  Constant6/1 -> Compare To Constant3/1
  Switch/1 -> Delay/1, flaps_applied/1
  [flap_control] -> If Action Subsystem4/2(last_flap_applied)
  [last_flap_applied] -> If Action Subsystem4/1(flap_control)
  AND3/1 -> If3/2
  AND2/1 -> If3/1
  att_sp_1/1 -> If Action Subsystem7/1(att_sp)
  [last_flaperons_applied] -> If Action Subsystem8/1(flaperon_control)
  In Bus Element/1 -> AND/1
  In Bus Element1/1 -> AND1/2
  In Bus Element3/1 -> AND2/1
  In Bus Element2/1 -> AND3/2
  AND/1 -> If/1
  AND1/1 -> If/2
  If/1 -> If Action Subsystem2/Action
  If/2 -> If Action Subsystem3/Action
  If Action Subsystem4/1(out) -> Switch/1
  Abs1/1 -> Switch/2
  [flap_control] -> Switch/3
  If Action Subsystem8/1(out) -> Switch1/1
  Abs/1 -> Switch1/2
  [flaperon_control] -> Switch1/3
  Switch1/1 -> Delay1/1, flaperons_applied/1

== system fw_att_control/Rate Control/Pitch Rate Controller ==
  pitch_bodyrate_setpoint : Inport
  ang_vel : Inport  Port=2
  Delay : Delay  DelayLength=1
  Saturation : Saturate  UpperLimit=1  LowerLimit=-1
      settings: AttributesFormatString=[%<LowerLimit>,%<UpperLimit>]
  Selector2 : Selector  InputPortWidth=3  IndexOptions=Index vector (dialog)  Indices=[2]  OutputSizes=1
  Sum : Sum  Inputs=+++
  Sum1 : Sum  Inputs=|+-
  前馈控制 : Subsystem
  比例控制 : Subsystem
  积分控制 : Subsystem
  pitch_u : Outport
  tag scope: pitch_last_output=global
  wires:
  Delay/1 -> [pitch_last_output]
  积分控制/1(out) -> Sum/3
  比例控制/1(out) -> Sum/2
  Sum1/1 -> 积分控制/1(pitch_rate_error), 比例控制/1(pitch_rate_error)  "pitch_rate_error"
  前馈控制/1(out) -> Sum/1
  pitch_bodyrate_setpoint/1 -> Sum1/1, 前馈控制/1(pitch_bodyrate_sp)
  Sum/1 -> Delay/1, Saturation/1
  ang_vel/1 -> Selector2/1
  Saturation/1 -> pitch_u/1  "pitch_u"
  Selector2/1 -> Sum1/2

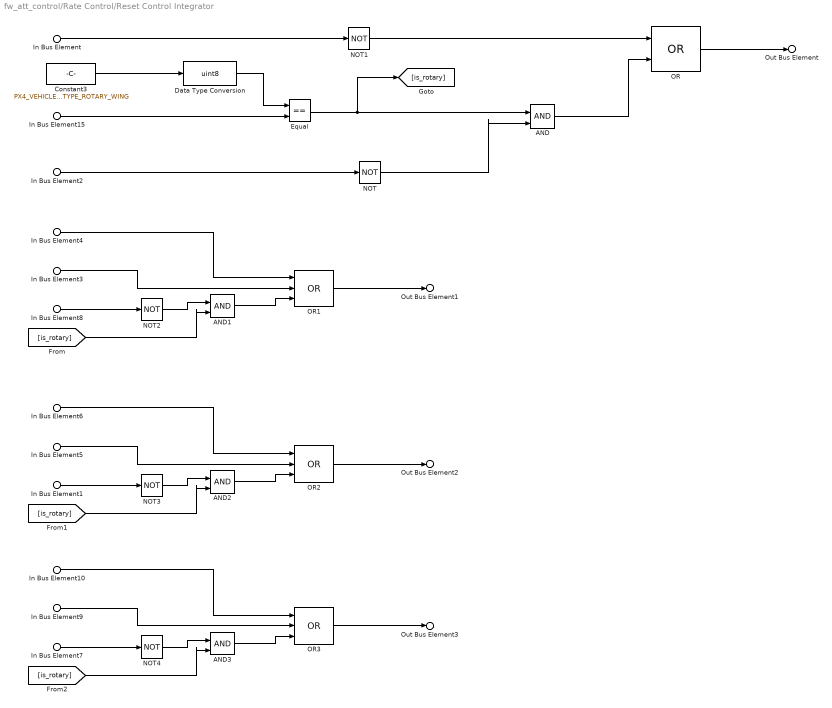
== system fw_att_control/Rate Control/Reset Control Integrator ==
  In Bus Element : Inport  PortName=vcontrol_mode  Element=flag_control_rates_enabled
  In Bus Element15 : Inport  Port=2  PortName=vehicle_status  Element=vehicle_type
  In Bus Element{1..2,7..8} (4 alike) : Inport  Port=2  PortName=vehicle_status  Element=in_transition_mode
  In Bus Element3 : Inport  Port=3  PortName=land_detected  Element=landed
  In Bus Element5 : Inport  Port=3  PortName=land_detected  Element=landed
  In Bus Element9 : Inport  Port=3  PortName=land_detected  Element=landed
  In Bus Element4 : Inport  Port=4  PortName=att_sp  Element=roll_reset_integral
  In Bus Element6 : Inport  Port=4  PortName=att_sp  Element=pitch_reset_integral
  In Bus Element10 : Inport  Port=4  PortName=att_sp  Element=yaw_reset_integral
  AND{,1..3} (4 alike) : Logic  IconShape=distinctive  AllPortsSameDT=off  OutDataTypeStr=boolean
  Constant3 : Constant  Value=PX4_VEHICLE_STATUS.VEHICLE_TYPE_ROTARY_WING
      settings: AttributesFormatString=%<Value>
  Data Type Conversion : DataTypeConversion  OutDataTypeStr=uint8
  Equal : RelationalOperator  Operator===  OutDataTypeStr=boolean  RndMeth=Simplest
  NOT{,1..4} (5 alike) : Logic  Operator=NOT  IconShape=distinctive  AllPortsSameDT=off  OutDataTypeStr=boolean
  OR : Logic  Operator=OR  IconShape=distinctive  AllPortsSameDT=off  OutDataTypeStr=boolean
  OR1 : Logic  Operator=OR  Inputs=3  IconShape=distinctive  AllPortsSameDT=off  OutDataTypeStr=boolean
  OR2 : Logic  Operator=OR  Inputs=3  IconShape=distinctive  AllPortsSameDT=off  OutDataTypeStr=boolean
  OR3 : Logic  Operator=OR  Inputs=3  IconShape=distinctive  AllPortsSameDT=off  OutDataTypeStr=boolean
  Out Bus Element : Outport  PortName=integrator_flag  Element=lock_integrator
  Out Bus Element1 : Outport  PortName=integrator_flag  Element=reset_roll_i
  Out Bus Element2 : Outport  PortName=integrator_flag  Element=reset_pitch_i
  Out Bus Element3 : Outport  PortName=integrator_flag  Element=reset_yaw_i
  wires:
  OR/1 -> Out Bus Element/1
  In Bus Element2/1 -> NOT/1
  In Bus Element/1 -> NOT1/1
  AND/1 -> OR/2
  OR1/1 -> Out Bus Element1/1
  In Bus Element8/1 -> NOT2/1
  Constant3/1 -> Data Type Conversion/1
  Data Type Conversion/1 -> Equal/1
  In Bus Element15/1 -> Equal/2
  Equal/1 -> [is_rotary], AND/1
  NOT2/1 -> AND1/1
  [is_rotary] -> AND1/2
  In Bus Element3/1 -> OR1/2
  In Bus Element4/1 -> OR1/1
  AND1/1 -> OR1/3
  AND2/1 -> OR2/3
  In Bus Element6/1 -> OR2/1
  In Bus Element5/1 -> OR2/2
  [is_rotary] -> AND2/2
  NOT3/1 -> AND2/1
  In Bus Element1/1 -> NOT3/1
  OR2/1 -> Out Bus Element2/1
  OR3/1 -> Out Bus Element3/1
  In Bus Element7/1 -> NOT4/1
  NOT4/1 -> AND3/1
  [is_rotary] -> AND3/2
  In Bus Element9/1 -> OR3/2
  In Bus Element10/1 -> OR3/1
  AND3/1 -> OR3/3
  NOT/1 -> AND/2
  NOT1/1 -> OR/1

== system fw_att_control/Rate Control/Roll Rate Controller ==
  roll_bodyrate_setpoint : Inport
  ang_vel : Inport  Port=2
  Delay : Delay  DelayLength=1
  Saturation : Saturate  UpperLimit=1  LowerLimit=-1
      settings: AttributesFormatString=[%<LowerLimit>,%<UpperLimit>]
  Selector1 : Selector  InputPortWidth=3  IndexOptions=Index vector (dialog)  Indices=[1]  OutputSizes=1
  Sum : Sum  Inputs=+++
  Sum1 : Sum  Inputs=|+-
  前馈控制 : Subsystem
  比例控制 : Subsystem
  积分控制 : Subsystem
  roll_u : Outport
  tag scope: roll_last_output=global
  wires:
  Sum/1 -> Delay/1, Saturation/1
  roll_bodyrate_setpoint/1 -> 前馈控制/1(roll_bodyrate_sp), Sum1/1
  前馈控制/1(out) -> Sum/1
  Sum1/1 -> 积分控制/1(roll_rate_error), 比例控制/1(roll_rate_error)  "roll_rate_error"
  比例控制/1(out) -> Sum/2
  积分控制/1(out) -> Sum/3
  Delay/1 -> [roll_last_output]
  ang_vel/1 -> Selector1/1
  Saturation/1 -> roll_u/1  "roll_u"
  Selector1/1 -> Sum1/2

== system fw_att_control/Rate Control/Wheel Rate Control ==
  yaw_bodyrate_setpoint : Inport
  ang_vel : Inport  Port=2
  Delay : Delay  DelayLength=1
  Saturation : Saturate  UpperLimit=1  LowerLimit=-1
      settings: AttributesFormatString=[%<LowerLimit>,%<UpperLimit>]
  Selector3 : Selector  InputPortWidth=3  IndexOptions=Index vector (dialog)  Indices=[3]  OutputSizes=1
  Sum : Sum  Inputs=|+-
  Sum1 : Sum  Inputs=+++
  前馈项 : Subsystem
  比例项 : Subsystem
  积分项 : Subsystem
  yaw_u : Outport
  tag scope: yaw_wheel_output=global
  wires:
  Sum1/1 -> Delay/1, Saturation/1
  ang_vel/1 -> Selector3/1
  Sum/1 -> 积分项/1(yaw_rate_error), 比例项/1(yaw_rate_error)  "yaw_rate_error"
  Selector3/1 -> Sum/2
  积分项/1(out) -> Sum1/3
  Delay/1 -> [yaw_wheel_output]
  yaw_bodyrate_setpoint/1 -> 前馈项/1(yaw_bodyrate_sp), Sum/1
  Saturation/1 -> yaw_u/1  "yaw_u"
  前馈项/1(out) -> Sum1/1
  比例项/1(out) -> Sum1/2

== system fw_att_control/Rate Control/Yaw Rate Control ==
  yaw_bodyrate_setpoint : Inport
  ang_vel : Inport  Port=2
  Delay : Delay  DelayLength=1
  Saturation : Saturate  UpperLimit=1  LowerLimit=-1  OutDataTypeStr=single
      settings: AttributesFormatString=[%<LowerLimit>,%<UpperLimit>]
  Selector4 : Selector  InputPortWidth=3  IndexOptions=Index vector (dialog)  Indices=[3]  OutputSizes=1
  Sum : Sum  Inputs=|+-
  Sum1 : Sum  Inputs=+++
  前馈项 : Subsystem
  比例项 : Subsystem
  积分项 : Subsystem
  yaw_u : Outport
  tag scope: yaw_last_output=global
  wires:
  Sum1/1 -> Delay/1, Saturation/1
  Sum/1 -> 比例项/1(yaw_rate_error), 积分项/1(yaw_rate_error)  "yaw_rate_error"
  积分项/1(out) -> Sum1/3
  Selector4/1 -> Sum/2
  yaw_bodyrate_setpoint/1 -> 前馈项/1(yaw_bodyrate_sp), Sum/1
  ang_vel/1 -> Selector4/1
  前馈项/1(out) -> Sum1/1
  比例项/1(out) -> Sum1/2
  Delay/1 -> [yaw_last_output]
  Saturation/1 -> yaw_u/1  "yaw_u"

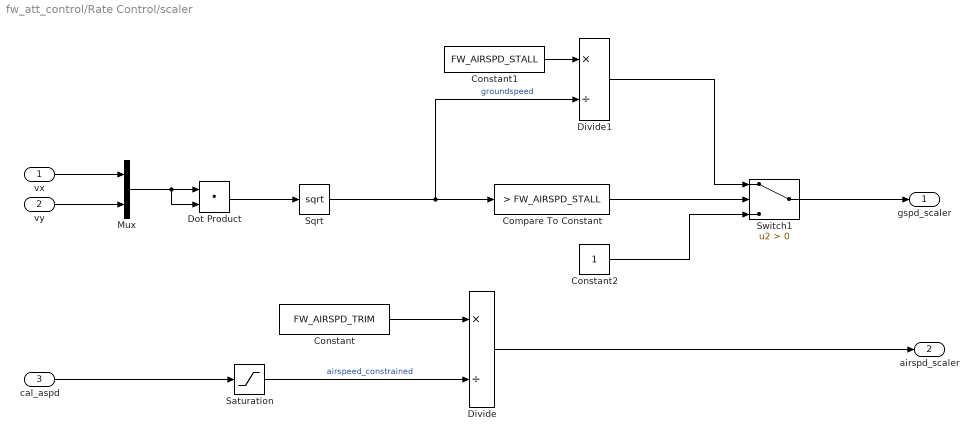
== system fw_att_control/Rate Control/scaler ==
  vx : Inport
  vy : Inport  Port=2
  cal_aspd : Inport  Port=3
  Compare To Constant : simulink/Logic and Bit Operations/Compare To Constant  relop=>  const=FW_AIRSPD_STALL  OutDataTypeStr=boolean
  Constant : Constant  Value=FW_AIRSPD_TRIM
  Constant1 : Constant  Value=FW_AIRSPD_STALL
  Constant2 : Constant  OutDataTypeStr=single
  Divide : Product  Inputs=*/
  Divide1 : Product  Inputs=*/
  Dot Product : DotProduct  InputSameDT=on  OutDataTypeStr=Inherit: Inherit via internal rule
  Mux : Mux  Inputs=2
  Saturation : Saturate  UpperLimit=FW_AIRSPD_MAX  LowerLimit=FW_AIRSPD_STALL
      settings: AttributesFormatString=[%<LowerLimit>,%<UpperLimit>]
  Sqrt : Sqrt  SaturateOnIntegerOverflow=on
  Switch1 : Switch  Criteria=u2 > Threshold
  gspd_scaler : Outport
  airspd_scaler : Outport  Port=2
  wires:
  Constant1/1 -> Divide1/1
  Mux/1 -> Dot Product/2, Dot Product/1
  Compare To Constant/1 -> Switch1/2
  Divide1/1 -> Switch1/1
  Sqrt/1 -> Divide1/2, Compare To Constant/1  "groundspeed"
  Constant2/1 -> Switch1/3
  Saturation/1 -> Divide/2  "airspeed_constrained"
  Dot Product/1 -> Sqrt/1
  Constant/1 -> Divide/1
  Switch1/1 -> gspd_scaler/1
  cal_aspd/1 -> Saturation/1
  Divide/1 -> airspd_scaler/1
  vx/1 -> Mux/1
  vy/1 -> Mux/2

== system fw_att_control/Auto Attitude Control/wheel control/Wrap -pi~pi ==
  In1 : Inport
  Constant1 : Constant  Value=2*pi  OutDataTypeStr=single
  Mod : Math  Operator=mod  SaturateOnIntegerOverflow=on
  Sum1 : Sum  Inputs=|+-
  Switch : Switch  Criteria=u2 > Threshold  Threshold=pi
  Out1 : Outport
  wires:
  Sum1/1 -> Switch/1
  Mod/1 -> Switch/3, Sum1/1, Switch/2
  Constant1/1 -> Sum1/2, Mod/2
  Switch/1 -> Out1/1
  In1/1 -> Mod/1

== system fw_att_control/Fix Control Yaw/Flaps Control/If Action Subsystem2 ==
  In Bus Element : Inport  PortName=man_control_sp  Element=flaps
  Action Port : ActionPort  ActionPortLabel=if(u1)
  Constant : Constant  OutDataTypeStr=single
  Gain : Gain  Gain=FW_FLAPS_SCL/2
  Sum : Sum  Inputs=|++
  flap_control : Outport
  wires:
  In Bus Element/1 -> Sum/1
  Constant/1 -> Sum/2
  Sum/1 -> Gain/1
  Gain/1 -> flap_control/1

== system fw_att_control/Fix Control Yaw/Flaps Control/If Action Subsystem3 ==
  In Bus Element1 : Inport  PortName=att_sp  Element=apply_flaps
  Action Port : ActionPort  ActionPortLabel=elseif(u2)
  Data Type Conversion : DataTypeConversion
  If Action Subsystem : Subsystem  TreatAsAtomicUnit=on
  If Action Subsystem1 : Subsystem  TreatAsAtomicUnit=on
  If Action Subsystem2 : Subsystem  TreatAsAtomicUnit=on
  Merge : Merge  Inputs=3
  Switch Case : SwitchCase  CaseConditions={0,1,2}  ShowDefaultCase=off
  out : Outport
  wires:
  Switch Case/1 -> If Action Subsystem/Action  "FLAPS_OFF"
  If Action Subsystem1/1(flap_control) -> Merge/2
  If Action Subsystem/1(flap_control) -> Merge/1
  Switch Case/2 -> If Action Subsystem1/Action  "FLAPS_LAND"
  Switch Case/3 -> If Action Subsystem2/Action  "FLAPS_TAKEOFF"
  If Action Subsystem2/1(flap_control) -> Merge/3
  Merge/1 -> out/1
  In Bus Element1/1 -> Data Type Conversion/1
  Data Type Conversion/1 -> Switch Case/1

== system fw_att_control/Fix Control Yaw/Flaps Control/If Action Subsystem4 ==
  flap_control : Inport
  last_flap_applied : Inport  Port=2
  Compare To Constant : simulink/Logic and Bit Operations/Compare To Constant  relop=<  const=0  OutDataTypeStr=boolean
  Sum : Sum  Inputs=|+-
  Switch : Switch  Criteria=u2 > Threshold
  Weighted Sample Time : SampleTimeMath
  Weighted Sample Time1 : SampleTimeMath  TsampMathOp=-
  last_flap_applied1 : InportShadow  Port=2
  last_flap_applied2 : InportShadow  Port=2
  out : Outport
  wires:
  last_flap_applied/1 -> Sum/1
  flap_control/1 -> Sum/2
  Sum/1 -> Compare To Constant/1
  Compare To Constant/1 -> Switch/2
  last_flap_applied2/1 -> Weighted Sample Time/1
  last_flap_applied1/1 -> Weighted Sample Time1/1
  Switch/1 -> out/1
  Weighted Sample Time/1 -> Switch/1
  Weighted Sample Time1/1 -> Switch/3

== system fw_att_control/Fix Control Yaw/Flaps Control/If Action Subsystem6 ==
  In Bus Element : Inport  PortName=man_control_sp  Element=aux2
  Action Port : ActionPort  ActionPortLabel=if(u1)
  Constant : Constant  OutDataTypeStr=single
  Gain : Gain  Gain=FW_FLAPERON_SCL/2
  Sum : Sum  Inputs=|++
  flaperon_control : Outport
  wires:
  In Bus Element/1 -> Sum/1
  Constant/1 -> Sum/2
  Sum/1 -> Gain/1
  Gain/1 -> flaperon_control/1

== system fw_att_control/Fix Control Yaw/Flaps Control/If Action Subsystem7 ==
  In Bus Element1 : Inport  PortName=att_sp  Element=apply_flaps
  Action Port : ActionPort  ActionPortLabel=elseif(u2)
  Constant : Constant  Value=PX4_VEHICLE_ATTITUDE_SETPOINT.FLAPS_LAND
      settings: AttributesFormatString=%<Value>
  Constant1 : Constant  Value=FW_FLAPERON_SCL  VectorParams1D=off
  Constant2 : Constant  Value=0  OutDataTypeStr=single
  Data Type Conversion : DataTypeConversion  OutDataTypeStr=uint8
  Equal : RelationalOperator  Operator===  OutDataTypeStr=boolean  RndMeth=Simplest
  Switch : Switch  Criteria=u2 > Threshold
  flaperon_control : Outport
  wires:
  Equal/1 -> Switch/2
  Constant1/1 -> Switch/1
  Constant2/1 -> Switch/3
  Switch/1 -> flaperon_control/1
  In Bus Element1/1 -> Equal/1
  Constant/1 -> Data Type Conversion/1
  Data Type Conversion/1 -> Equal/2

== system fw_att_control/Fix Control Yaw/Flaps Control/If Action Subsystem8 ==
  flaperon_control : Inport
  last_flaperons_applied : Inport  Port=2
  Compare To Constant : simulink/Logic and Bit Operations/Compare To Constant  relop=<  const=0  OutDataTypeStr=boolean
  Sum : Sum  Inputs=|+-
  Switch : Switch  Criteria=u2 > Threshold
  Weighted Sample Time : SampleTimeMath  TsampMathOp=-
  Weighted Sample Time1 : SampleTimeMath
  last_flap_applied1 : InportShadow  Port=2
  last_flap_applied3 : InportShadow  Port=2
  out : Outport
  wires:
  last_flaperons_applied/1 -> Sum/1
  flaperon_control/1 -> Sum/2
  Sum/1 -> Compare To Constant/1
  Compare To Constant/1 -> Switch/2
  Switch/1 -> out/1
  last_flap_applied1/1 -> Weighted Sample Time/1
  last_flap_applied3/1 -> Weighted Sample Time1/1
  Weighted Sample Time1/1 -> Switch/1
  Weighted Sample Time/1 -> Switch/3

== system fw_att_control/Rate Control/Pitch Rate Controller/前馈控制 ==
  pitch_bodyrate_sp : Inport
  Gain : Gain  Gain=FW_RR_FF
  Product : Product
  out : Outport
  wires:
  Product/1 -> out/1
  pitch_bodyrate_sp/1 -> Gain/1
  Gain/1 -> Product/2
  [airspd_scaler] -> Product/1

== system fw_att_control/Rate Control/Pitch Rate Controller/比例控制 ==
  pitch_rate_error : Inport
  Gain1 : Gain  Gain=FW_PR_P
  Math Function1 : Math  Operator=magnitude^2  SaturateOnIntegerOverflow=on
  Product2 : Product
  out : Outport
  wires:
  Product2/1 -> out/1
  pitch_rate_error/1 -> Gain1/1
  Gain1/1 -> Product2/2
  Math Function1/1 -> Product2/1
  [airspd_scaler] -> Math Function1/1

== system fw_att_control/Rate Control/Pitch Rate Controller/积分控制 ==
  pitch_rate_error : Inport
  Abs : Abs
  Bus Selector : BusSelector  OutputSignals=lock_integrator
  Bus Selector1 : BusSelector  OutputSignals=reset_pitch_i
  Compare To Constant : simulink/Logic and Bit Operations/Compare To Constant  relop=>  const=1  OutDataTypeStr=boolean
  Constant : Constant  Value=0  OutDataTypeStr=single
  Discrete-Time Integrator : DiscreteIntegrator  gainval=FW_RR_I  ExternalReset=level  SampleTime=-1  LimitOutput=on  UpperSaturationLimit=FW_PR_IMAX  LowerSaturationLimit=-FW_PR_IMAX  ICPrevOutput=DiscIntNeverNeededParam  ICPrevScaledInput=DiscIntNeverNeededParam
  Math Function1 : Math  Operator=magnitude^2  SaturateOnIntegerOverflow=on
  NOT : Logic  Operator=NOT  IconShape=distinctive  AllPortsSameDT=off  OutDataTypeStr=boolean
  Product : Product  Inputs=3
  Switch : Switch  Criteria=u2 > Threshold
  out : Outport
  wires:
  pitch_rate_error/1 -> Product/2
  Math Function1/1 -> Product/3
  NOT/1 -> Product/1
  Discrete-Time Integrator/1 -> out/1
  [airspd_scaler] -> Math Function1/1
  [integrator_flag] -> Bus Selector/1
  Bus Selector/1 -> NOT/1  "<lock_integrator>"
  [integrator_flag] -> Bus Selector1/1
  Bus Selector1/1 -> Discrete-Time Integrator/2  "<reset_pitch_i>"
  [pitch_last_output] -> Abs/1
  Abs/1 -> Compare To Constant/1
  Compare To Constant/1 -> Switch/2
  Constant/1 -> Switch/1
  Product/1 -> Switch/3  "pitch_id"
  Switch/1 -> Discrete-Time Integrator/1

== system fw_att_control/Rate Control/Roll Rate Controller/前馈控制 ==
  roll_bodyrate_sp : Inport
  Gain : Gain  Gain=FW_RR_FF
  Product : Product
  out : Outport
  wires:
  Gain/1 -> Product/2
  roll_bodyrate_sp/1 -> Gain/1
  Product/1 -> out/1
  [airspd_scaler] -> Product/1

== system fw_att_control/Rate Control/Roll Rate Controller/比例控制 ==
  roll_rate_error : Inport
  Gain1 : Gain  Gain=FW_PR_P
  Math Function1 : Math  Operator=magnitude^2  SaturateOnIntegerOverflow=on
  Product2 : Product
  out : Outport
  wires:
  Math Function1/1 -> Product2/1
  Gain1/1 -> Product2/2
  roll_rate_error/1 -> Gain1/1
  Product2/1 -> out/1
  [airspd_scaler] -> Math Function1/1

== system fw_att_control/Rate Control/Roll Rate Controller/积分控制 ==
  roll_rate_error : Inport
  Abs : Abs
  Bus Selector : BusSelector  OutputSignals=lock_integrator
  Bus Selector1 : BusSelector  OutputSignals=reset_roll_i
  Compare To Constant : simulink/Logic and Bit Operations/Compare To Constant  relop=>  const=1  OutDataTypeStr=boolean
  Constant : Constant  Value=0  OutDataTypeStr=single
  Discrete-Time Integrator : DiscreteIntegrator  gainval=FW_RR_I  ExternalReset=level  SampleTime=-1  LimitOutput=on  UpperSaturationLimit=FW_PR_IMAX  LowerSaturationLimit=-FW_PR_IMAX  ICPrevOutput=DiscIntNeverNeededParam  ICPrevScaledInput=DiscIntNeverNeededParam
  Math Function1 : Math  Operator=magnitude^2  SaturateOnIntegerOverflow=on
  NOT : Logic  Operator=NOT  IconShape=distinctive  AllPortsSameDT=off  OutDataTypeStr=boolean
  Product : Product  Inputs=3
  Switch : Switch  Criteria=u2 > Threshold
  out : Outport
  wires:
  Discrete-Time Integrator/1 -> out/1
  NOT/1 -> Product/1
  Math Function1/1 -> Product/3
  roll_rate_error/1 -> Product/2
  [airspd_scaler] -> Math Function1/1
  [integrator_flag] -> Bus Selector/1
  Bus Selector/1 -> NOT/1  "<lock_integrator>"
  [integrator_flag] -> Bus Selector1/1
  Bus Selector1/1 -> Discrete-Time Integrator/2  "<reset_roll_i>"
  [roll_last_output] -> Abs/1
  Abs/1 -> Compare To Constant/1
  Compare To Constant/1 -> Switch/2
  Constant/1 -> Switch/1
  Product/1 -> Switch/3  "roll_id"
  Switch/1 -> Discrete-Time Integrator/1

== system fw_att_control/Rate Control/Wheel Rate Control/前馈项 ==
  yaw_bodyrate_sp : Inport
  Gain : Gain  Gain=FW_WR_FF
  Product : Product
  out : Outport
  wires:
  yaw_bodyrate_sp/1 -> Gain/1
  Product/1 -> out/1
  Gain/1 -> Product/2
  [gspd_scaler] -> Product/1

== system fw_att_control/Rate Control/Wheel Rate Control/比例项 ==
  yaw_rate_error : Inport
  Gain2 : Gain  Gain=FW_WR_P
  Math Function : Math  Operator=magnitude^2  SaturateOnIntegerOverflow=on
  Product : Product
  out : Outport
  wires:
  yaw_rate_error/1 -> Gain2/1
  Math Function/1 -> Product/1
  Gain2/1 -> Product/2
  Product/1 -> out/1
  [gspd_scaler] -> Math Function/1
